simulink model "MSD_parest_sim_sol"  (R2023b)
settings: Solver=ode3  StartTime=0.0  StopTime=200  FixedStep=0.01  RelTol=1e-3
values from neighbouring files (symbols this model uses):
  A_F = A-B*K    [MSD_parest_par_sol.m]
  B_F = [ 0 ; 0 ; -A_F(3,1)]    [MSD_parest_par_sol.m]
  C_F0 = [ 1 0 0 ]    [MSD_parest_par_sol.m]
  C_F1 = [ 0 1 0 ]    [MSD_parest_par_sol.m]
  C_F2 = [ 0 0 1 ]    [MSD_parest_par_sol.m]
  d = 0.1    [MSD_parest_par_sol.m]    (also in d_pend_par_sol.m)
  k = 5    [MSD_parest_par_sol.m]
  m = 10    [MSD_parest_par_sol.m]    (also in d_pend_par_sol.m = 50)
  theta = [ a0 ; a1 ; b ]    [MSD_parest_par_sol.m]
settings Model: Creator=jerome  LastModifiedBy=jerome
settings ModelReferenceCC: EnableRefExpFcnMdlSchedulingChecks=on

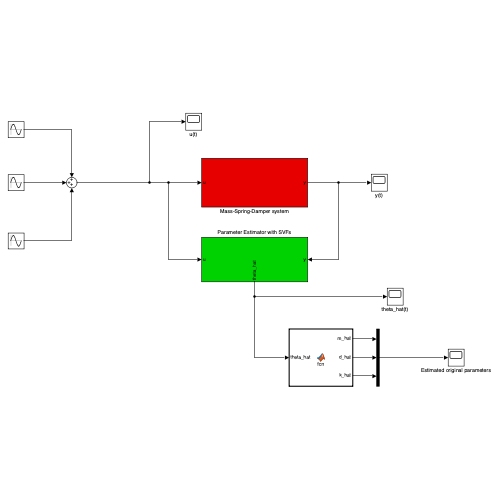
[thumbnail: Simulink's stored preview of the top-level diagram]
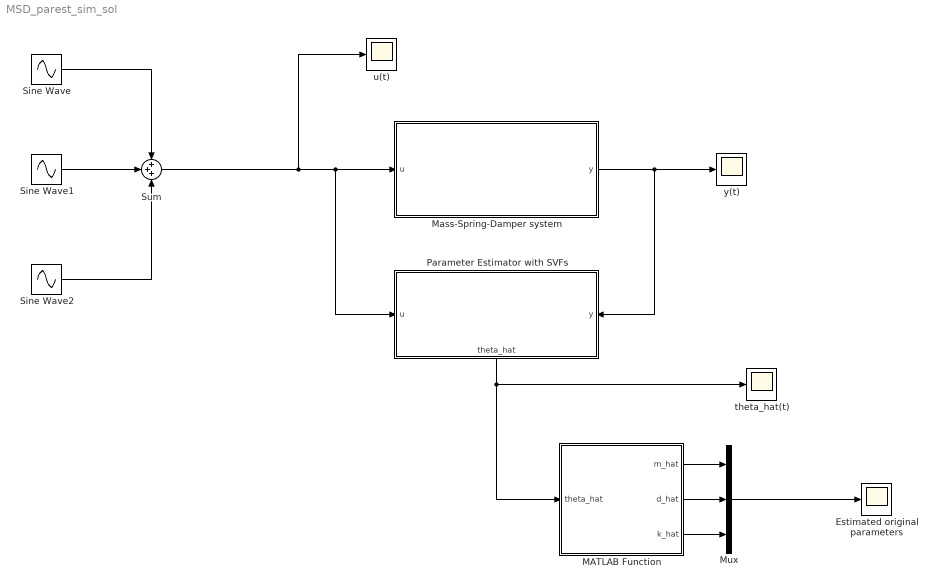
== system MSD_parest_sim_sol ==
  Estimated original parameters : Scope
  MATLAB Function : MATLAB Function  TreatAsAtomicUnit=on
  Mass-Spring-Damper system : Subsystem
  Mux : Mux  Inputs=3
  Parameter Estimator with SVFs : Subsystem
      settings: PortSchema="{\"entries\":[{\"content\":{\"sides\":[{\"content\":{\"connectorIds\":[\"In1\"]},\"type\":\"ConnectorPlacement.EquallySpacedRectSide\",\"uuid\":\"701dba22-d81c-4620-a4f9-4eedebec699b\"},{\"content\":{\"connectorIds\":[\"In2\"],\"side\":\"RIGHT\"},\"type\":\"ConnectorPlacement.EquallySpacedRectSide\",\"uuid\":\"14a753f7-073c-4e1b-870d-b975b59fa292\"},{\"content\":{\"connectorIds\":[],\"side\":\"TOP\"},\"type\":\"ConnectorPlacement.EquallySpacedRectSide\",\"uuid\":\"4fae71d8-e84c-4ac4-80a0-9291851fcc8b\"},{\"content\":{\"connectorIds\":[\"Out1\"],\"side\":\"BOTTOM\"},\"type\":\"ConnectorPlacement.EquallySpacedRectSide\",\"uuid\":\"a05140d0-bc49-4091-9e05-f62f82fd2c00\"}]},\"type\":\"ConnectorPlacement.EquallySpacedConnector\",\"uuid\":\"49c9441c-c785-42d3-a441-16a536410442\"}],\"packageUris\":[\"http://schema.mathworks.com/mf0/Connector/R2020b\"],\"version\":\"1.0\"}"
  Sine Wave : Sin  Phase=pi*rand  SampleTime=0
  Sine Wave1 : Sin  Frequency=2  Phase=pi/5  SampleTime=0
  Sine Wave2 : Sin  Frequency=0.5  Phase=pi/3  SampleTime=0
  Sum : Sum  Inputs=+++
  theta_hat(t) : Scope
  u(t) : Scope
  y(t) : Scope
  wires:
  Mass-Spring-Damper system/1(y) -> Parameter Estimator with SVFs/2(y), y(t)/1
  Sum/1 -> u(t)/1, Parameter Estimator with SVFs/1(u), Mass-Spring-Damper system/1(u)
  Sine Wave/1 -> Sum/1
  Sine Wave1/1 -> Sum/2
  Sine Wave2/1 -> Sum/3
  Parameter Estimator with SVFs/1(theta_hat) -> theta_hat(t)/1, MATLAB Function/1(theta_hat)
  MATLAB Function/2(d_hat) -> Mux/2
  MATLAB Function/1(m_hat) -> Mux/1
  MATLAB Function/3(k_hat) -> Mux/3
  Mux/1 -> Estimated original parameters/1

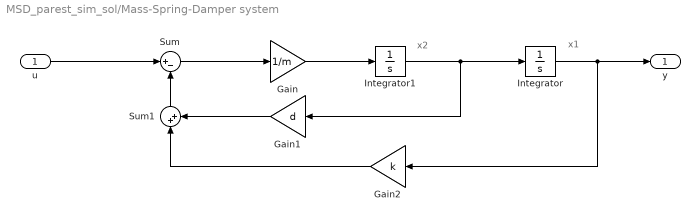
== system MSD_parest_sim_sol/Mass-Spring-Damper system ==
  note: x2
  note: x1
  u : Inport
  Gain : Gain  Gain=1/m
  Gain1 : Gain  Gain=d
  Gain2 : Gain  Gain=k
  Integrator : Integrator
  Integrator1 : Integrator
  Sum : Sum  Inputs=|+-
  Sum1 : Sum  Inputs=|++
  y : Outport
  wires:
  Integrator/1 -> Gain2/1, y/1
  Integrator1/1 -> Gain1/1, Integrator/1
  u/1 -> Sum/1
  Gain/1 -> Integrator1/1
  Sum/1 -> Gain/1
  Gain1/1 -> Sum1/2
  Sum1/1 -> Sum/2
  Gain2/1 -> Sum1/1

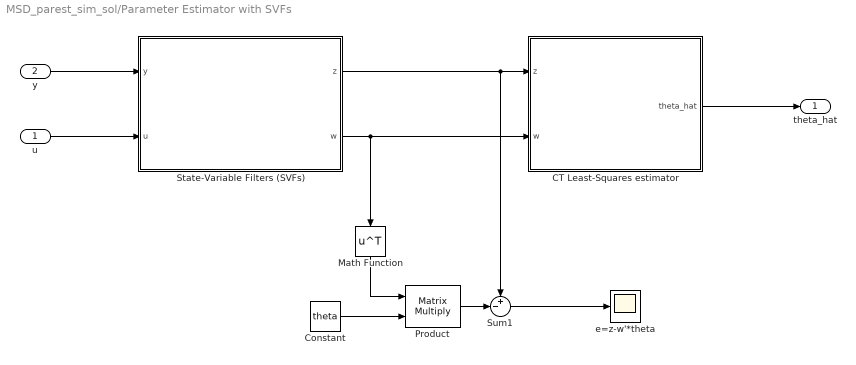
== system MSD_parest_sim_sol/Parameter Estimator with SVFs ==
  u : Inport
  y : Inport  Port=2
  CT Least-Squares estimator : Subsystem
  Constant : Constant  Value=theta  VectorParams1D=off
  Math Function : Math  Operator=transpose
  Product : Product  Multiplication=Matrix(*)
  State-Variable Filters (SVFs) : Subsystem
  Sum1 : Sum  Inputs=+-|
  e=z-w'*theta : Scope
  theta_hat : Outport
  wires:
  CT Least-Squares estimator/1(theta_hat) -> theta_hat/1
  State-Variable Filters (SVFs)/1(z) -> Sum1/1, CT Least-Squares estimator/1(z)
  State-Variable Filters (SVFs)/2(w) -> CT Least-Squares estimator/2(w), Math Function/1
  y/1 -> State-Variable Filters (SVFs)/1(y)
  u/1 -> State-Variable Filters (SVFs)/2(u)
  Constant/1 -> Product/2
  Product/1 -> Sum1/2
  Math Function/1 -> Product/1
  Sum1/1 -> e=z-w'*theta/1

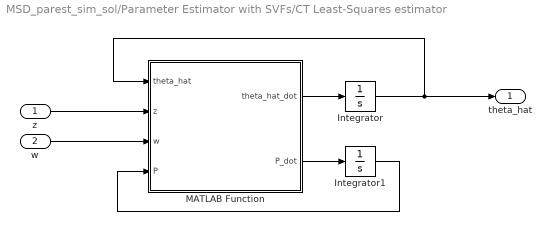
== system MSD_parest_sim_sol/Parameter Estimator with SVFs/CT Least-Squares estimator ==
  z : Inport
  w : Inport  Port=2
  Integrator : Integrator  InitialCondition=zeros(3,1)
  Integrator1 : Integrator  InitialCondition=1000*eye(3)
  MATLAB Function : MATLAB Function  TreatAsAtomicUnit=on
  theta_hat : Outport
  wires:
  z/1 -> MATLAB Function/2(z)
  w/1 -> MATLAB Function/3(w)
  MATLAB Function/1(theta_hat_dot) -> Integrator/1
  Integrator1/1 -> MATLAB Function/4(P)
  Integrator/1 -> theta_hat/1, MATLAB Function/1(theta_hat)
  MATLAB Function/2(P_dot) -> Integrator1/1

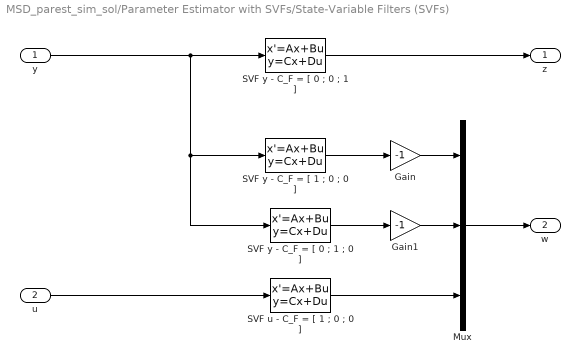
== system MSD_parest_sim_sol/Parameter Estimator with SVFs/State-Variable Filters (SVFs) ==
  y : Inport
  u : Inport  Port=2
  Gain : Gain  Gain=-1
  Gain1 : Gain  Gain=-1
  Mux : Mux  Inputs=3
  SVF u - C_F = [ 1 ; 0 ; 0 ] : StateSpace  A=A_F  B=B_F  C=C_F0  D=0  InitialCondition=zeros(3,1)
  SVF y - C_F = [ 0 ; 0 ; 1 ] : StateSpace  A=A_F  B=B_F  C=C_F2  D=0  InitialCondition=ones(3,1)
  SVF y - C_F = [ 0 ; 1 ; 0 ] : StateSpace  A=A_F  B=B_F  C=C_F1  D=0  InitialCondition=zeros(3,1)
  SVF y - C_F = [ 1 ; 0 ; 0 ] : StateSpace  A=A_F  B=B_F  C=C_F0  D=0  InitialCondition=zeros(3,1)
  z : Outport
  w : Outport  Port=2
  wires:
  SVF y - C_F = [ 0 ; 0 ; 1 ]/1 -> z/1
  u/1 -> SVF u - C_F = [ 1 ; 0 ; 0 ]/1
  SVF y - C_F = [ 1 ; 0 ; 0 ]/1 -> Gain/1
  Gain1/1 -> Mux/2
  Mux/1 -> w/1
  y/1 -> SVF y - C_F = [ 1 ; 0 ; 0 ]/1, SVF y - C_F = [ 0 ; 1 ; 0 ]/1, SVF y - C_F = [ 0 ; 0 ; 1 ]/1
  SVF u - C_F = [ 1 ; 0 ; 0 ]/1 -> Mux/3
  Gain/1 -> Mux/1
  SVF y - C_F = [ 0 ; 1 ; 0 ]/1 -> Gain1/1

== matlab function MSD_parest_sim_sol/Parameter Estimator with SVFs/CT Least-Squares estimator/MATLAB Function ==
  data: theta_hat input; theta_hat_dot output; P_dot output; z input; w input; P input
function [theta_hat_dot,P_dot] = fcn(theta_hat,z,w,P)

%theta_hat_dot = P*w*(z - w'*theta_hat);
%P_dot = -P*w*w'*P;

% normalized version
theta_hat_dot = P*w/(1+w'*P*w)*(z - w'*theta_hat);
P_dot = -P*w*w'/(1+w'*P*w)*P;

== matlab function MSD_parest_sim_sol/MATLAB Function ==
  data: theta_hat input; m_hat output; d_hat output; k_hat output
function [m_hat,d_hat,k_hat] = fcn(theta_hat)

a0_hat = theta_hat(1);
a1_hat = theta_hat(2);
b_hat = theta_hat(3);

if abs(b_hat)<= 0.01 % to avoid singularities
    m_hat = 0;
    d_hat = 0;
    k_hat = 0;
else 
    m_hat = 1/b_hat;
    d_hat = a1_hat * m_hat;
    k_hat = a0_hat * m_hat;
end
